simulink model "simpSimuRoboToGoNurAbstandPD"  (R2019b)
settings: Solver=ode45  StartTime=0.0  StopTime=150.0  RelTol=1e-3  EnableMultiTasking=on
libraries: roblocks x1, simulink x1
settings Model: Creator=pic  LastModifiedBy=mackst
settings SolverCC: ZeroCrossAlgorithm=Adaptive
settings DataIOCC: SaveFormat=Array  TimeSaveName=t  OutputSaveName=y
settings OptimizationCC: ExpressionDepthLimit=2147483647  LifeSpan=inf
settings DebuggingCC: UnderspecifiedInitializationDetection=Classic  MergeDetectMultiDrivingBlocksExec=none  IgnoredZcDiagnostic=none  SolverPrmCheckMsg=warning  AllowSymbolicDim=off  StateNameClashWarn=warning  SFUnexpectedBacktrackingDiag=warning  SFNoUnconditionalDefaultTransitionDiag=warning  SFExecutionAtInitializationDiag=none  ArithmeticOperatorsInVariantConditions=warning
settings HardwareCC: ProdBitPerPointer=32  ProdBitPerSizeT=32  ProdBitPerPtrDiffT=32  ProdLargestAtomicFloat=None  ProdIntDivRoundTo=Undefined  ProdEndianess=Unspecified  ProdWordSize=32  ProdHWDeviceType=32-bit Generic
settings ModelReferenceCC: PropagateSignalLabelsOutOfModel=off
settings SFSimCC: SimUseLocalCustomCode=off  CustomCodeUndefinedFunction=UseInterfaceOnly
settings RTWCC: RTWUseLocalCustomCode=off
settings CodeAppCC: StateflowObjectComments=on
settings GRTTargetCC: TargetLangStandard=C89/C90 (ANSI)  GeneratePreprocessorConditionals=Disable all  CombineOutputUpdateFcns=off  GRTInterface=on
settings ConfigComp: CovMetricSettings=dw  CovHtmlReporting=on  CovSaveCumulativeToWorkspaceVar=on  CovSaveSingleToWorkspaceVar=on  CovExternalEMLEnable=off

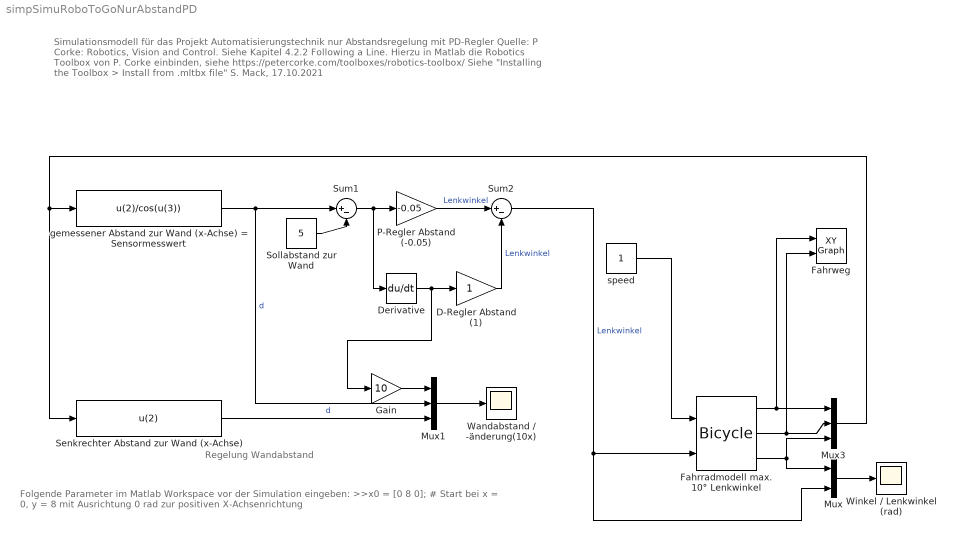
== system simpSimuRoboToGoNurAbstandPD ==
  note: Folgende Parameter im Matlab Workspace vor der Simulation eingeben:
      | >>x0 = [0 8 0]; # Start bei x = 0, y = 8 mit Ausrichtung 0 rad zur positiven X-Achsenrichtung
  note: Regelung Wandabstand
  note: Simulationsmodell für das Projekt Automatisierungstechnik nur Abstandsregelung mit PD-Regler
      | Quelle: P Corke: Robotics, Vision and Control. Siehe Kapitel 4.2.2 Following a Line.
      |
      | Hierzu in Matlab die Robotics Toolbox von P. Corke einbinden, siehe https://petercorke.com/toolboxes/robotics-toolbox/
      | Siehe "Installing the Toolbox > Install from .mltbx file"
      |
      | S. Mack, 17.10.2021
  D-Regler Abstand (1) : Gain
  Derivative : Derivative
  Fahrradmodell max. 10° Lenkwinkel : roblocks/Vehicles/Bicycle  vlim=0.4  accel=1  alim=0.05  steer_rate=Inf  L=1  x0=x0
  Fahrweg : simulink/Sinks/XY Graph  xmin=0  xmax=100  ymin=0  ymax=10  st=-1
  Gain : Gain  Gain=10
  Mux : Mux  Inputs=2
  Mux1 : Mux  Inputs=3
  Mux3 : Mux  Inputs=3
  P-Regler Abstand (-0.05) : Gain  Gain=-0.05
  Senkrechter Abstand zur Wand (x-Achse) : Fcn  Expr=u(2)
  Sollabstand zur Wand : Constant  Value=5
  Sum1 : Sum  Inputs=|+-
  Sum2 : Sum  Inputs=|+-
  Wandabstand / -änderung(10x) : Scope
  Winkel / Lenkwinkel (rad) : Scope
  gemessener Abstand zur Wand (x-Achse) = Sensormesswert : Fcn  Expr=u(2)/cos(u(3))
  speed : Constant  VectorParams1D=off  SampleTime=0.02
  wires:
  Mux3/1 -> Senkrechter Abstand zur Wand (x-Achse)/1, gemessener Abstand zur Wand (x-Achse) = Sensormesswert/1
  speed/1 -> Fahrradmodell max. 10° Lenkwinkel/1
  Sum2/1 -> Mux/2, Fahrradmodell max. 10° Lenkwinkel/2  "Lenkwinkel"
  Fahrradmodell max. 10° Lenkwinkel/1 -> Fahrweg/1, Mux3/1
  Fahrradmodell max. 10° Lenkwinkel/2 -> Fahrweg/2, Mux3/2
  Fahrradmodell max. 10° Lenkwinkel/3 -> Mux/1, Mux3/3
  Sum1/1 -> Derivative/1, P-Regler Abstand (-0.05)/1
  Sollabstand zur Wand/1 -> Sum1/2
  Mux1/1 -> Wandabstand / -änderung(10x)/1
  gemessener Abstand zur Wand (x-Achse) = Sensormesswert/1 -> Mux1/2, Sum1/1  "d"
  Senkrechter Abstand zur Wand (x-Achse)/1 -> Mux1/3  "d"
  Mux/1 -> Winkel / Lenkwinkel (rad)/1
  Derivative/1 -> Gain/1, D-Regler Abstand (1)/1
  P-Regler Abstand (-0.05)/1 -> Sum2/1  "Lenkwinkel"
  D-Regler Abstand (1)/1 -> Sum2/2  "Lenkwinkel"
  Gain/1 -> Mux1/1
